simulink model "EX_Relay_1"  (Simulink 8.4)
settings: Solver=ode45  StartTime=0.0  StopTime=2  MaxStep=0.001  RelTol=1e-3
libraries: simulink x1
settings Model: Creator=kiril_000  LastModifiedBy=kiril_000
settings OptimizationCC: BooleanDataType=off  ExpressionDepthLimit=128
settings DebuggingCC: SaveWithParameterizedLinksMsg=none  SignalResolutionControl=TryResolveAllWithWarning  SolverPrmCheckMsg=none  MultiTaskDSMMsg=warning  MultiTaskCondExecSysMsg=none  FcnCallInpInsideContextMsg=EnableAllAsError  StateNameClashWarn=none
settings HardwareCC: TargetUnknown=on
settings RTWCC: IncludeERTFirstTime=on

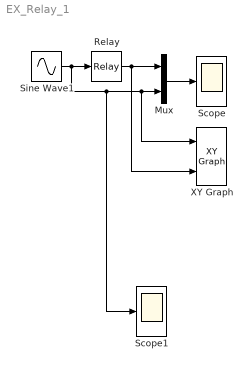
== system EX_Relay_1 ==
  Mux : Mux  Inputs=2
  Relay : Relay  OnSwitchValue=0.5  OffSwitchValue=-0.5  OffOutputValue=-1
  Scope : Scope
      settings: TimeRange=2  YMin=-1.1  YMax=1.1
  Scope1 : Scope
      settings: TimeRange=2  YMin=-1  YMax=-0.4
  Sine Wave1 : Sin  Frequency=6.28  SampleTime=0
  XY Graph : simulink/Sinks/XY Graph  xmin=-1.1  xmax=1.1  ymin=-1.1  ymax=1.1  st=-1
  wires:
  Sine Wave1/1 -> Scope1/1, Mux/2, XY Graph/1, Relay/1
  Mux/1 -> Scope/1
  Relay/1 -> Mux/1, XY Graph/2
